simulink model "chap5_1sim"  (Simulink 8.1)
settings: Solver=ode45  StartTime=0.0  StopTime=100  FixedStep=0.001  RelTol=1e-3
settings Model: Creator=ljk  LastModifiedBy=liujk  ExtModeTrigMode=oneshot  ExtModeArmWhenConnect=off
settings DataIOCC: LimitDataPoints=off  SignalLoggingName=sigsOut
settings OptimizationCC: BooleanDataType=off
settings DebuggingCC: SaveWithParameterizedLinksMsg=none  SignalResolutionControl=TryResolveAllWithWarning  SolverPrmCheckMsg=none  MultiTaskDSMMsg=warning  MultiTaskCondExecSysMsg=none  StrictBusMsg=None
settings HardwareCC: TargetUnknown=on
settings RTWCC: IncludeERTFirstTime=on

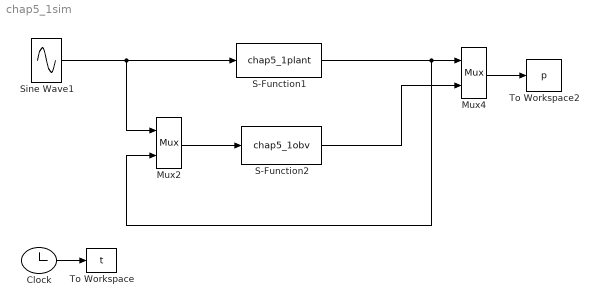
== system chap5_1sim ==
  Clock : Clock
  Mux2 : Mux  Inputs=2
  Mux4 : Mux  Inputs=2
  S-Function1 : S-Function  FunctionName=chap5_1plant  EnableBusSupport=off
  S-Function2 : S-Function  FunctionName=chap5_1obv  EnableBusSupport=off
  Sine Wave1 : Sin  Frequency=100  SampleTime=0
  To Workspace : ToWorkspace  VariableName=t  SampleTime=-1
  To Workspace2 : ToWorkspace  VariableName=p  SampleTime=-1
  wires:
  S-Function1/1 -> Mux2/2, Mux4/1
  Clock/1 -> To Workspace/1
  Mux4/1 -> To Workspace2/1
  Sine Wave1/1 -> Mux2/1, S-Function1/1
  S-Function2/1 -> Mux4/2
  Mux2/1 -> S-Function2/1
